simulink model "PPG_sensor_module"  (R2023a)
settings: Solver=FixedStepDiscrete  StartTime=0.0  StopTime=60  FixedStep=1/300  RelTol=1e-3
libraries: arduinolib x1
settings Model: Creator=Ananya  LastModifiedBy=Ananya
settings OptimizationCC: DefaultParameterBehavior=Inlined  EnhancedBackFolding=on  PassReuseOutputArgsAs=Individual arguments  ZeroExternalMemoryAtStartup=off  ZeroInternalMemoryAtStartup=off  MaxStackSize=64  OptimizeBlockOrder=speed  DifferentSizesBufferReuse=on  OptimizationCustomize=off  EfficientTunableParamExpr=on
settings DebuggingCC: ParameterTunabilityLossMsg=error  UnconnectedInputMsg=warning  UnconnectedOutputMsg=warning  UnconnectedLineMsg=warning
settings HardwareCC: ProdBitPerInt=16  ProdBitPerPointer=16  ProdBitPerSizeT=16  ProdBitPerPtrDiffT=16  ProdLargestAtomicFloat=None  ProdWordSize=8  ProdHWDeviceType=Atmel->AVR
settings ModelReferenceCC: EnableRefExpFcnMdlSchedulingChecks=on
settings SFSimCC: MATLABDynamicMemAlloc=off
settings RTWCC: Description=Embedded Coder  SystemTargetFile=ert.tlc  TemplateMakefile=ert_default_tmf  Toolchain=Arduino AVR  BuildConfiguration=Faster Runs  DLArmComputeVersion=19.05
settings CodeAppCC: ForceParamTrailComments=on  IgnoreCustomStorageClasses=off  OperatorAnnotations=on  SimulinkDataObjDesc=on  SFDataObjDesc=on  InsertBlockDesc=on
settings ERTTargetCC: SupportContinuousTime=on  ExtModeTransport=3  ExtModeStaticAlloc=on  ExtModeStaticAllocSize=2048  ExtModeMexFile=ext_xcp  ExtModeIntrfLevel=Level2 - Open  ERTCustomFileTemplate=example_file_process.tlc

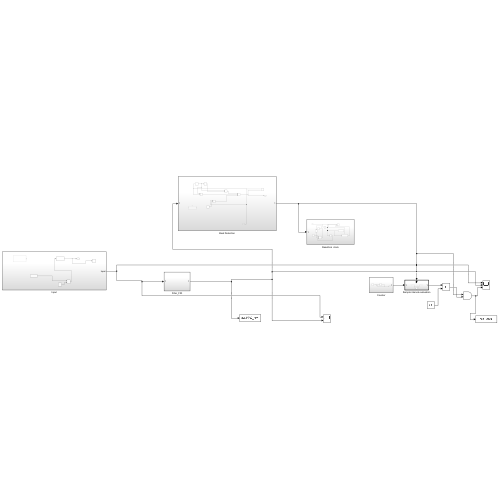
[thumbnail: Simulink's stored preview of the top-level diagram]
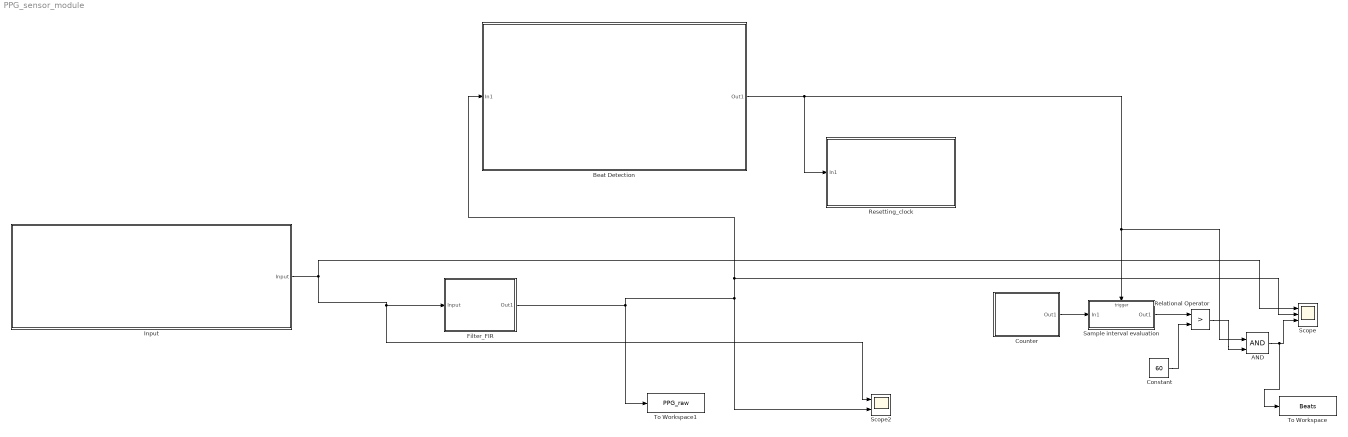
== system PPG_sensor_module ==
  AND : Logic  IconShape=distinctive  AllPortsSameDT=off  OutDataTypeStr=boolean
  Beat Detection : Subsystem
  Constant : Constant  Value=60  OutDataTypeStr=int16
  Counter : Subsystem
  Filter_FIR : Subsystem  Tag=FilterWizardSubSystem
      settings: ErrorFcn=dspFilterRealizedInBasicElemsAlgLoopErrFcnCallback
  Input : Subsystem
  Relational Operator : RelationalOperator  Operator=>  OutDataTypeStr=boolean  RndMeth=Simplest  InputSameDT=off
  Resetting_clock : Subsystem
  Sample interval evaluation : Subsystem  TreatAsAtomicUnit=on
  Scope : Scope  NumInputPorts=3
  Scope2 : Scope  NumInputPorts=2
  To Workspace : ToWorkspace  VariableName=Beats  SaveFormat=Timeseries  SampleTime=-1
  To Workspace1 : ToWorkspace  VariableName=PPG_raw  SaveFormat=Timeseries  SampleTime=-1
  wires:
  Counter/1(Out1) -> Sample interval evaluation/1(In1)
  AND/1 -> To Workspace/1, Scope/3
  Input/1(Input) -> Scope/1, Scope2/1, Filter_FIR/1(Input)
  Constant/1 -> Relational Operator/2
  Sample interval evaluation/1(Out1) -> Relational Operator/1
  Relational Operator/1 -> AND/2
  Filter_FIR/1(Out1) -> To Workspace1/1, Scope2/2, Beat Detection/1(In1), Scope/2
  Beat Detection/1(Out1) -> Resetting_clock/1(In1), AND/1, Sample interval evaluation/Trigger

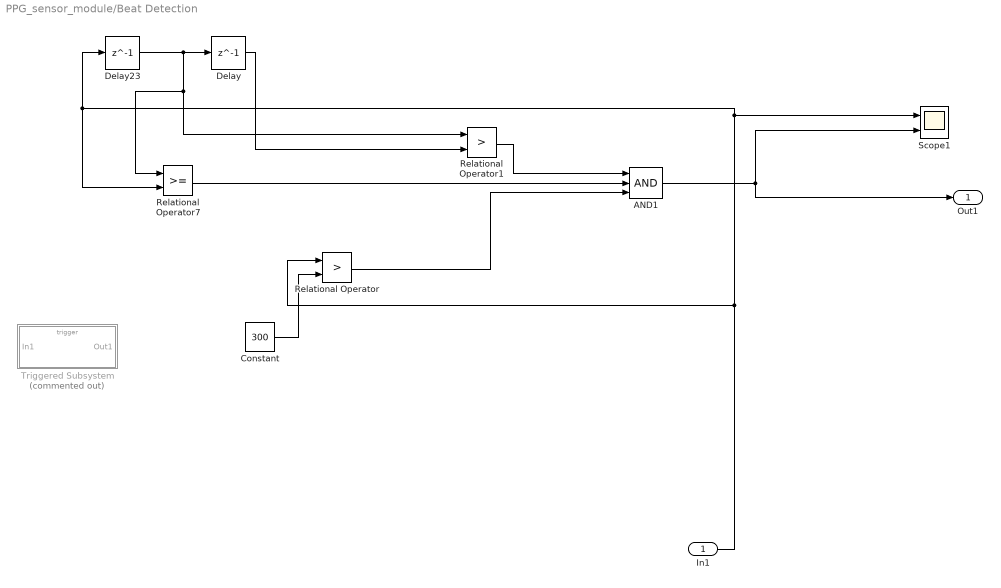
== system PPG_sensor_module/Beat Detection ==
  In1 : Inport
  AND1 : Logic  Inputs=3  IconShape=distinctive  AllPortsSameDT=off  OutDataTypeStr=boolean
  Constant : Constant  Value=300
  Delay : Delay  DelayLength=1
  Delay23 : Delay  DelayLength=1
  Relational Operator : RelationalOperator  Operator=>  OutDataTypeStr=boolean  RndMeth=Simplest  InputSameDT=off
  Relational Operator1 : RelationalOperator  Operator=>  OutDataTypeStr=boolean  RndMeth=Simplest  InputSameDT=off
  Relational Operator7 : RelationalOperator  OutDataTypeStr=boolean  RndMeth=Simplest  InputSameDT=off
  Scope1 : Scope  NumInputPorts=2
  Triggered Subsystem : Subsystem  Commented=on  TreatAsAtomicUnit=on
  Out1 : Outport
  wires:
  AND1/1 -> Scope1/2, Out1/1
  Relational Operator1/1 -> AND1/1
  Delay23/1 -> Relational Operator1/1, Relational Operator7/1, Delay/1
  In1/1 -> Relational Operator/1, Relational Operator7/2, Delay23/1, Scope1/1
  Relational Operator7/1 -> AND1/2
  Delay/1 -> Relational Operator1/2
  Constant/1 -> Relational Operator/2
  Relational Operator/1 -> AND1/3

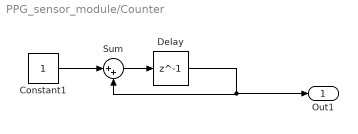
== system PPG_sensor_module/Counter ==
  Constant1 : Constant  OutDataTypeStr=int16
  Delay : Delay  DelayLength=1
  Sum : Sum  Inputs=|++
  Out1 : Outport
  wires:
  Delay/1 -> Out1/1, Sum/2
  Constant1/1 -> Sum/1
  Sum/1 -> Delay/1

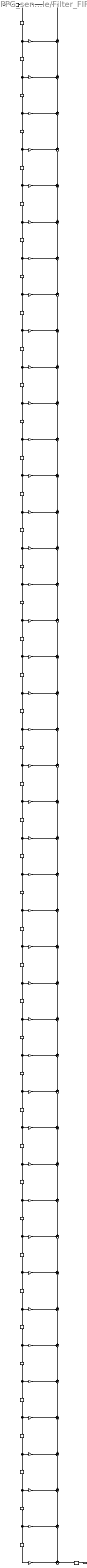
== system PPG_sensor_module/Filter_FIR ==
  Input : Inport
  BodyDelay{2..44} (43 alike) : Delay  DelayLength=1  InitialCondition=0
  BodyLSum{2..44} (43 alike) : Sum  Inputs=++|  AccumDataTypeStr=fixdt(1,35,23)  OutDataTypeStr=fixdt(1,35,23)  RndMeth=Convergent
  ConvertIn : DataTypeConversion  OutDataTypeStr=fixdt(1,16,5)  RndMeth=Nearest
  ConvertOut : DataTypeConversion  OutDataTypeStr=fixdt(1,35,23)  RndMeth=Convergent  SaturateOnIntegerOverflow=off
  b(1) : Gain  Gain=0.00179703366251263868  ParamDataTypeStr=fixdt(1,16,18)  OutDataTypeStr=fixdt(1,31,23)  RndMeth=Convergent
  b(10) : Gain  Gain=-0.0107693714306029576  ParamDataTypeStr=fixdt(1,16,18)  OutDataTypeStr=fixdt(1,31,23)  RndMeth=Convergent
  b(11) : Gain  Gain=-0.00596573994074645585  ParamDataTypeStr=fixdt(1,16,18)  OutDataTypeStr=fixdt(1,31,23)  RndMeth=Convergent
  b(12) : Gain  Gain=0.000775060719917803048  ParamDataTypeStr=fixdt(1,16,18)  OutDataTypeStr=fixdt(1,31,23)  RndMeth=Convergent
  b(13) : Gain  Gain=0.00936342771953894287  ParamDataTypeStr=fixdt(1,16,18)  OutDataTypeStr=fixdt(1,31,23)  RndMeth=Convergent
  b(14) : Gain  Gain=0.0195519814208151704  ParamDataTypeStr=fixdt(1,16,18)  OutDataTypeStr=fixdt(1,31,23)  RndMeth=Convergent
  b(15) : Gain  Gain=0.0309451334419993361  ParamDataTypeStr=fixdt(1,16,18)  OutDataTypeStr=fixdt(1,31,23)  RndMeth=Convergent
  b(16) : Gain  Gain=0.0430177062034670654  ParamDataTypeStr=fixdt(1,16,18)  OutDataTypeStr=fixdt(1,31,23)  RndMeth=Convergent
  b(17) : Gain  Gain=0.0551469400629030077  ParamDataTypeStr=fixdt(1,16,18)  OutDataTypeStr=fixdt(1,31,23)  RndMeth=Convergent
  b(18) : Gain  Gain=0.0666554673554519694  ParamDataTypeStr=fixdt(1,16,18)  OutDataTypeStr=fixdt(1,31,23)  RndMeth=Convergent
  b(19) : Gain  Gain=0.0768652920623881658  ParamDataTypeStr=fixdt(1,16,18)  OutDataTypeStr=fixdt(1,31,23)  RndMeth=Convergent
  b(2) : Gain  Gain=-0.00736331124644262237  ParamDataTypeStr=fixdt(1,16,18)  OutDataTypeStr=fixdt(1,31,23)  RndMeth=Convergent
  b(20) : Gain  Gain=0.08515066374523661  ParamDataTypeStr=fixdt(1,16,18)  OutDataTypeStr=fixdt(1,31,23)  RndMeth=Convergent
  b(21) : Gain  Gain=0.090989227298761674  ParamDataTypeStr=fixdt(1,16,18)  OutDataTypeStr=fixdt(1,31,23)  RndMeth=Convergent
  b(22) : Gain  Gain=0.0940061121572491332  ParamDataTypeStr=fixdt(1,16,18)  OutDataTypeStr=fixdt(1,31,23)  RndMeth=Convergent
  b(23) : Gain  Gain=0.0940061121572491332  ParamDataTypeStr=fixdt(1,16,18)  OutDataTypeStr=fixdt(1,31,23)  RndMeth=Convergent
  b(24) : Gain  Gain=0.090989227298761674  ParamDataTypeStr=fixdt(1,16,18)  OutDataTypeStr=fixdt(1,31,23)  RndMeth=Convergent
  b(25) : Gain  Gain=0.08515066374523661  ParamDataTypeStr=fixdt(1,16,18)  OutDataTypeStr=fixdt(1,31,23)  RndMeth=Convergent
  b(26) : Gain  Gain=0.0768652920623881658  ParamDataTypeStr=fixdt(1,16,18)  OutDataTypeStr=fixdt(1,31,23)  RndMeth=Convergent
  b(27) : Gain  Gain=0.0666554673554519694  ParamDataTypeStr=fixdt(1,16,18)  OutDataTypeStr=fixdt(1,31,23)  RndMeth=Convergent
  b(28) : Gain  Gain=0.0551469400629030077  ParamDataTypeStr=fixdt(1,16,18)  OutDataTypeStr=fixdt(1,31,23)  RndMeth=Convergent
  b(29) : Gain  Gain=0.0430177062034670654  ParamDataTypeStr=fixdt(1,16,18)  OutDataTypeStr=fixdt(1,31,23)  RndMeth=Convergent
  b(3) : Gain  Gain=-0.00717579044660151752  ParamDataTypeStr=fixdt(1,16,18)  OutDataTypeStr=fixdt(1,31,23)  RndMeth=Convergent
  b(30) : Gain  Gain=0.0309451334419993361  ParamDataTypeStr=fixdt(1,16,18)  OutDataTypeStr=fixdt(1,31,23)  RndMeth=Convergent
  b(31) : Gain  Gain=0.0195519814208151704  ParamDataTypeStr=fixdt(1,16,18)  OutDataTypeStr=fixdt(1,31,23)  RndMeth=Convergent
  b(32) : Gain  Gain=0.00936342771953894287  ParamDataTypeStr=fixdt(1,16,18)  OutDataTypeStr=fixdt(1,31,23)  RndMeth=Convergent
  b(33) : Gain  Gain=0.000775060719917803048  ParamDataTypeStr=fixdt(1,16,18)  OutDataTypeStr=fixdt(1,31,23)  RndMeth=Convergent
  b(34) : Gain  Gain=-0.00596573994074645585  ParamDataTypeStr=fixdt(1,16,18)  OutDataTypeStr=fixdt(1,31,23)  RndMeth=Convergent
  b(35) : Gain  Gain=-0.0107693714306029576  ParamDataTypeStr=fixdt(1,16,18)  OutDataTypeStr=fixdt(1,31,23)  RndMeth=Convergent
  b(36) : Gain  Gain=-0.0136903881325173352  ParamDataTypeStr=fixdt(1,16,18)  OutDataTypeStr=fixdt(1,31,23)  RndMeth=Convergent
  b(37) : Gain  Gain=-0.0149102626624502219  ParamDataTypeStr=fixdt(1,16,18)  OutDataTypeStr=fixdt(1,31,23)  RndMeth=Convergent
  b(38) : Gain  Gain=-0.0147084768212589825  ParamDataTypeStr=fixdt(1,16,18)  OutDataTypeStr=fixdt(1,31,23)  RndMeth=Convergent
  b(39) : Gain  Gain=-0.0134309063069368018  ParamDataTypeStr=fixdt(1,16,18)  OutDataTypeStr=fixdt(1,31,23)  RndMeth=Convergent
  b(4) : Gain  Gain=-0.00914242226961629878  ParamDataTypeStr=fixdt(1,16,18)  OutDataTypeStr=fixdt(1,31,23)  RndMeth=Convergent
  b(40) : Gain  Gain=-0.011440304918506063  ParamDataTypeStr=fixdt(1,16,18)  OutDataTypeStr=fixdt(1,31,23)  RndMeth=Convergent
  b(41) : Gain  Gain=-0.00914242226961629878  ParamDataTypeStr=fixdt(1,16,18)  OutDataTypeStr=fixdt(1,31,23)  RndMeth=Convergent
  b(42) : Gain  Gain=-0.00717579044660151752  ParamDataTypeStr=fixdt(1,16,18)  OutDataTypeStr=fixdt(1,31,23)  RndMeth=Convergent
  b(43) : Gain  Gain=-0.00736331124644262237  ParamDataTypeStr=fixdt(1,16,18)  OutDataTypeStr=fixdt(1,31,23)  RndMeth=Convergent
  b(44) : Gain  Gain=0.00179703366251263868  ParamDataTypeStr=fixdt(1,16,18)  OutDataTypeStr=fixdt(1,31,23)  RndMeth=Convergent
  b(5) : Gain  Gain=-0.011440304918506063  ParamDataTypeStr=fixdt(1,16,18)  OutDataTypeStr=fixdt(1,31,23)  RndMeth=Convergent
  b(6) : Gain  Gain=-0.0134309063069368018  ParamDataTypeStr=fixdt(1,16,18)  OutDataTypeStr=fixdt(1,31,23)  RndMeth=Convergent
  b(7) : Gain  Gain=-0.0147084768212589825  ParamDataTypeStr=fixdt(1,16,18)  OutDataTypeStr=fixdt(1,31,23)  RndMeth=Convergent
  b(8) : Gain  Gain=-0.0149102626624502219  ParamDataTypeStr=fixdt(1,16,18)  OutDataTypeStr=fixdt(1,31,23)  RndMeth=Convergent
  b(9) : Gain  Gain=-0.0136903881325173352  ParamDataTypeStr=fixdt(1,16,18)  OutDataTypeStr=fixdt(1,31,23)  RndMeth=Convergent
  Out1 : Outport
  wires:
  Input/1 -> ConvertIn/1
  b(1)/1 -> BodyLSum2/2
  ConvertIn/1 -> b(1)/1, BodyDelay2/1
  BodyDelay2/1 -> b(2)/1, BodyDelay3/1
  b(2)/1 -> BodyLSum2/1
  BodyLSum2/1 -> BodyLSum3/2
  BodyDelay3/1 -> b(3)/1, BodyDelay4/1
  b(3)/1 -> BodyLSum3/1
  BodyLSum3/1 -> BodyLSum4/2
  BodyDelay4/1 -> b(4)/1, BodyDelay5/1
  b(4)/1 -> BodyLSum4/1
  BodyLSum4/1 -> BodyLSum5/2
  BodyDelay5/1 -> b(5)/1, BodyDelay6/1
  b(5)/1 -> BodyLSum5/1
  BodyLSum5/1 -> BodyLSum6/2
  BodyDelay6/1 -> b(6)/1, BodyDelay7/1
  b(6)/1 -> BodyLSum6/1
  BodyLSum6/1 -> BodyLSum7/2
  BodyDelay7/1 -> b(7)/1, BodyDelay8/1
  b(7)/1 -> BodyLSum7/1
  BodyLSum7/1 -> BodyLSum8/2
  BodyDelay8/1 -> b(8)/1, BodyDelay9/1
  b(8)/1 -> BodyLSum8/1
  BodyLSum8/1 -> BodyLSum9/2
  BodyDelay9/1 -> b(9)/1, BodyDelay10/1
  b(9)/1 -> BodyLSum9/1
  BodyLSum9/1 -> BodyLSum10/2
  BodyDelay10/1 -> b(10)/1, BodyDelay11/1
  b(10)/1 -> BodyLSum10/1
  BodyLSum10/1 -> BodyLSum11/2
  BodyDelay11/1 -> b(11)/1, BodyDelay12/1
  b(11)/1 -> BodyLSum11/1
  BodyLSum11/1 -> BodyLSum12/2
  BodyDelay12/1 -> b(12)/1, BodyDelay13/1
  b(12)/1 -> BodyLSum12/1
  BodyLSum12/1 -> BodyLSum13/2
  BodyDelay13/1 -> b(13)/1, BodyDelay14/1
  b(13)/1 -> BodyLSum13/1
  BodyLSum13/1 -> BodyLSum14/2
  BodyDelay14/1 -> b(14)/1, BodyDelay15/1
  b(14)/1 -> BodyLSum14/1
  BodyLSum14/1 -> BodyLSum15/2
  BodyDelay15/1 -> b(15)/1, BodyDelay16/1
  b(15)/1 -> BodyLSum15/1
  BodyLSum15/1 -> BodyLSum16/2
  BodyDelay16/1 -> b(16)/1, BodyDelay17/1
  b(16)/1 -> BodyLSum16/1
  BodyLSum16/1 -> BodyLSum17/2
  BodyDelay17/1 -> b(17)/1, BodyDelay18/1
  b(17)/1 -> BodyLSum17/1
  BodyLSum17/1 -> BodyLSum18/2
  BodyDelay18/1 -> b(18)/1, BodyDelay19/1
  b(18)/1 -> BodyLSum18/1
  BodyLSum18/1 -> BodyLSum19/2
  BodyDelay19/1 -> b(19)/1, BodyDelay20/1
  b(19)/1 -> BodyLSum19/1
  BodyLSum19/1 -> BodyLSum20/2
  BodyDelay20/1 -> b(20)/1, BodyDelay21/1
  b(20)/1 -> BodyLSum20/1
  BodyLSum20/1 -> BodyLSum21/2
  BodyDelay21/1 -> b(21)/1, BodyDelay22/1
  b(21)/1 -> BodyLSum21/1
  BodyLSum21/1 -> BodyLSum22/2
  BodyDelay22/1 -> b(22)/1, BodyDelay23/1
  b(22)/1 -> BodyLSum22/1
  BodyLSum22/1 -> BodyLSum23/2
  BodyDelay23/1 -> b(23)/1, BodyDelay24/1
  b(23)/1 -> BodyLSum23/1
  BodyLSum23/1 -> BodyLSum24/2
  BodyDelay24/1 -> b(24)/1, BodyDelay25/1
  b(24)/1 -> BodyLSum24/1
  BodyLSum24/1 -> BodyLSum25/2
  BodyDelay25/1 -> b(25)/1, BodyDelay26/1
  b(25)/1 -> BodyLSum25/1
  BodyLSum25/1 -> BodyLSum26/2
  BodyDelay26/1 -> b(26)/1, BodyDelay27/1
  b(26)/1 -> BodyLSum26/1
  BodyLSum26/1 -> BodyLSum27/2
  BodyDelay27/1 -> b(27)/1, BodyDelay28/1
  b(27)/1 -> BodyLSum27/1
  BodyLSum27/1 -> BodyLSum28/2
  BodyDelay28/1 -> b(28)/1, BodyDelay29/1
  b(28)/1 -> BodyLSum28/1
  BodyLSum28/1 -> BodyLSum29/2
  BodyDelay29/1 -> b(29)/1, BodyDelay30/1
  b(29)/1 -> BodyLSum29/1
  BodyLSum29/1 -> BodyLSum30/2
  BodyDelay30/1 -> b(30)/1, BodyDelay31/1
  b(30)/1 -> BodyLSum30/1
  BodyLSum30/1 -> BodyLSum31/2
  BodyDelay31/1 -> b(31)/1, BodyDelay32/1
  b(31)/1 -> BodyLSum31/1
  BodyLSum31/1 -> BodyLSum32/2
  BodyDelay32/1 -> b(32)/1, BodyDelay33/1
  b(32)/1 -> BodyLSum32/1
  BodyLSum32/1 -> BodyLSum33/2
  BodyDelay33/1 -> b(33)/1, BodyDelay34/1
  b(33)/1 -> BodyLSum33/1
  BodyLSum33/1 -> BodyLSum34/2
  BodyDelay34/1 -> b(34)/1, BodyDelay35/1
  b(34)/1 -> BodyLSum34/1
  BodyLSum34/1 -> BodyLSum35/2
  BodyDelay35/1 -> b(35)/1, BodyDelay36/1
  b(35)/1 -> BodyLSum35/1
  BodyLSum35/1 -> BodyLSum36/2
  BodyDelay36/1 -> b(36)/1, BodyDelay37/1
  b(36)/1 -> BodyLSum36/1
  BodyLSum36/1 -> BodyLSum37/2
  BodyDelay37/1 -> b(37)/1, BodyDelay38/1
  b(37)/1 -> BodyLSum37/1
  BodyLSum37/1 -> BodyLSum38/2
  BodyDelay38/1 -> b(38)/1, BodyDelay39/1
  b(38)/1 -> BodyLSum38/1
  BodyLSum38/1 -> BodyLSum39/2
  BodyDelay39/1 -> b(39)/1, BodyDelay40/1
  b(39)/1 -> BodyLSum39/1
  BodyLSum39/1 -> BodyLSum40/2
  BodyDelay40/1 -> b(40)/1, BodyDelay41/1
  b(40)/1 -> BodyLSum40/1
  BodyLSum40/1 -> BodyLSum41/2
  BodyDelay41/1 -> b(41)/1, BodyDelay42/1
  b(41)/1 -> BodyLSum41/1
  BodyLSum41/1 -> BodyLSum42/2
  BodyDelay42/1 -> b(42)/1, BodyDelay43/1
  b(42)/1 -> BodyLSum42/1
  BodyLSum42/1 -> BodyLSum43/2
  BodyDelay43/1 -> b(43)/1, BodyDelay44/1
  b(43)/1 -> BodyLSum43/1
  BodyLSum43/1 -> BodyLSum44/1
  BodyDelay44/1 -> b(44)/1
  b(44)/1 -> BodyLSum44/2
  BodyLSum44/1 -> ConvertOut/1
  ConvertOut/1 -> Out1/1

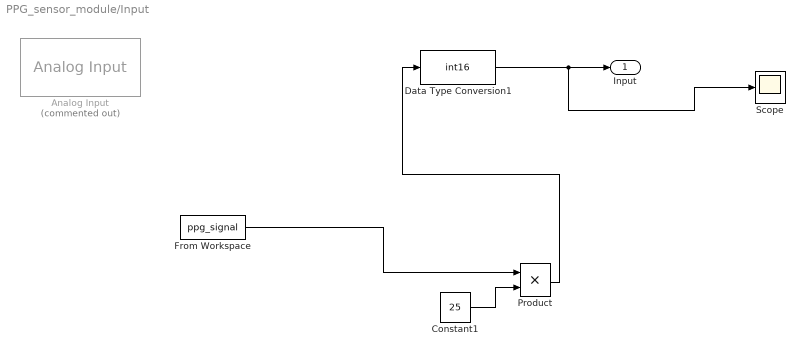
== system PPG_sensor_module/Input ==
  Analog Input : arduinolib/Analog Input  Commented=on  pinNumber=0  ReadResultsOnly=off  ConversionTriggerSource=Software  ExternalTriggerType=uint32( 0 )  OutputDataType=uint16  EnableConversionCompleteNotify=off  EnableOuputStatus=off  SampleTime=-1  blockPlatform=arduino
  Constant1 : Constant  Value=25  OutDataTypeStr=uint16
  Data Type Conversion1 : DataTypeConversion  OutDataTypeStr=int16  SaturateOnIntegerOverflow=off  RndMeth=Floor
  From Workspace : FromWorkspace  VariableName=ppg_signal
  Product : Product
  Scope : Scope
  Input : Outport
  wires:
  Constant1/1 -> Product/2
  Data Type Conversion1/1 -> Scope/1, Input/1
  From Workspace/1 -> Product/1
  Product/1 -> Data Type Conversion1/1

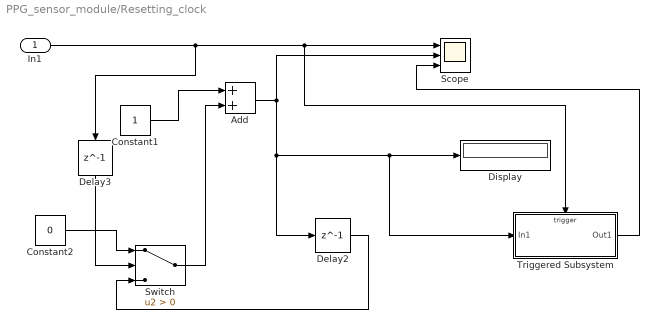
== system PPG_sensor_module/Resetting_clock ==
  In1 : Inport
  Add : Sum  OutDataTypeStr=int16
  Constant1 : Constant  OutDataTypeStr=int16
  Constant2 : Constant  Value=0
  Delay2 : Delay  DelayLength=1  InitialCondition=-1
  Delay3 : Delay  DelayLength=1
  Display : Display
  Scope : Scope  NumInputPorts=3
  Switch : Switch  Criteria=u2 > Threshold  OutDataTypeStr=int16  SaturateOnIntegerOverflow=off  InputSameDT=off
  Triggered Subsystem : Subsystem  TreatAsAtomicUnit=on
  wires:
  Add/1 -> Triggered Subsystem/1(In1), Display/1, Delay2/1, Scope/2
  Constant2/1 -> Switch/1
  Switch/1 -> Add/2
  Triggered Subsystem/1(Out1) -> Scope/3
  In1/1 -> Delay3/1, Triggered Subsystem/Trigger, Scope/1
  Delay2/1 -> Switch/3
  Constant1/1 -> Add/1
  Delay3/1 -> Switch/2

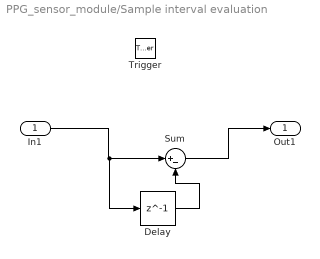
== system PPG_sensor_module/Sample interval evaluation ==
  In1 : Inport
  Trigger : TriggerPort  VariantControl=(inherit)
  Delay : Delay  DelayLength=1
  Sum : Sum  Inputs=|+-
  Out1 : Outport
  wires:
  In1/1 -> Delay/1, Sum/1
  Sum/1 -> Out1/1
  Delay/1 -> Sum/2

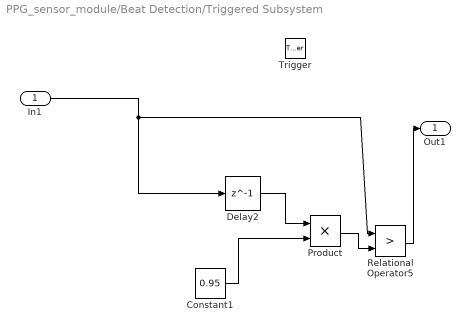
== system PPG_sensor_module/Beat Detection/Triggered Subsystem ==
  In1 : Inport
  Trigger : TriggerPort  VariantControl=(inherit)
  Constant1 : Constant  Value=0.95
  Delay2 : Delay  DelayLength=1
  Product : Product
  Relational Operator5 : RelationalOperator  Operator=>  OutDataTypeStr=boolean  RndMeth=Simplest  InputSameDT=off
  Out1 : Outport
  wires:
  Product/1 -> Relational Operator5/2
  Constant1/1 -> Product/2
  Delay2/1 -> Product/1
  Relational Operator5/1 -> Out1/1
  In1/1 -> Relational Operator5/1, Delay2/1

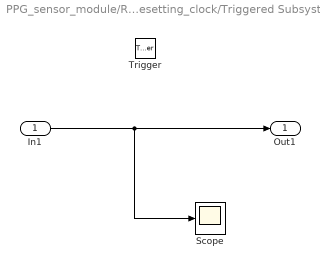
== system PPG_sensor_module/Resetting_clock/Triggered Subsystem ==
  In1 : Inport
  Trigger : TriggerPort  VariantControl=(inherit)
  Scope : Scope
  Out1 : Outport
  wires:
  In1/1 -> Scope/1, Out1/1
